simulink model "Ejercicio8"  (R2020a)
settings: Solver=ode15s  StartTime=0.0  StopTime=15  MaxStep=0.012  RelTol=1e-3
values from neighbouring files (symbols this model uses):
  c = 2000    [Ejercicio7_parametros.m]    (also in Ejercicio8_parametros.m)
  k1 = 22000    [Ejercicio8_parametros.m]
  k2 = 10000    [Ejercicio8_parametros.m]
  m1 = 250    [Ejercicio8_parametros.m]
  m2 = 25    [Ejercicio8_parametros.m]
libraries: fl_lib x10, nesl_utility x6, SignalEditorBlockLib x1, sdl_lib x1
settings Model: Creator=juan  LastModifiedBy=juan

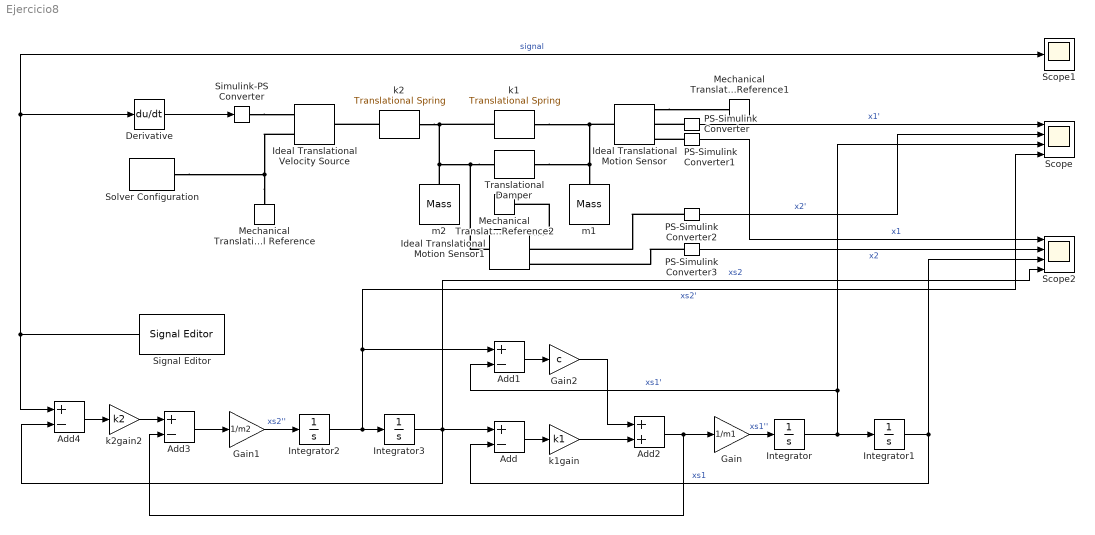
== system Ejercicio8 ==
  Add{,1,3..4} (4 alike) : Sum  Inputs=+-
  Add2 : Sum
  Derivative : Derivative
  Gain : Gain  Gain=1/m1
  Gain1 : Gain  Gain=1/m2
  Gain2 : Gain  Gain=c
  Ideal Translational Motion Sensor : fl_lib/Mechanical/Mechanical Sensors/Ideal Translational Motion Sensor  offset=0 m
  Ideal Translational Motion Sensor1 : fl_lib/Mechanical/Mechanical Sensors/Ideal Translational Motion Sensor  offset=0 m
  Ideal Translational Velocity Source : fl_lib/Mechanical/Mechanical Sources/Ideal Translational Velocity Source
  Integrator{,1..3} (4 alike) : Integrator
  Mechanical Translational Reference : fl_lib/Mechanical/Translational Elements/Mechanical Translational Reference
  Mechanical Translational Reference1 : fl_lib/Mechanical/Translational Elements/Mechanical Translational Reference
  Mechanical Translational Reference2 : fl_lib/Mechanical/Translational Elements/Mechanical Translational Reference
  PS-Simulink Converter{,1..3} (4 alike) : nesl_utility/PS-Simulink Converter  PhysicalDomain=network_engine_domain  SubClassName=ps_output  LeftPortType=input  RightPortType=output  PseudoPeriodic=off  Frequencies=[]  Unit=inherit  AffineConversion=off
  Scope : Scope  NumInputPorts=4
  Scope1 : Scope
  Scope2 : Scope  NumInputPorts=4
  Signal Editor : SignalEditorBlockLib/Signal Editor  FileName=Ejercicio7_terreno.mat  ActiveScenario=Scenario  ActiveSignal=Signal 1  IsBus=off  OutputBusObjectStr=Bus: BusObject  SampleTime=0  ZeroCross=off  OutputAfterFinalValue=Setting to zero  Unit=inherit  PreserveSignalName=on
  Simulink-PS Converter : nesl_utility/Simulink-PS Converter  PhysicalDomain=network_engine_domain  SubClassName=ps_input  LeftPortType=input  RightPortType=output  PseudoPeriodic=off  Frequencies=[]  NoiseDistribution=none  NoiseParameters=[]  Unit=1  AffineConversion=off  FilteringAndDerivatives=provide  SimscapeFilterOrder=1  InputFilterTimeConstant=0.001  UdotUserProvided=0
  Solver Configuration : nesl_utility/Solver Configuration  PhysicalDomain=network_engine_domain  SubClassName=solver  LeftPortType=input  RightPortType=generic  Tones=[]  Harmonics=[]  SimulateNoise=off  Profile=off  UseLocalSampling=off  EnableSwitchedLinearOptims=on  FrequencyDomain=off  UseCCode=off  RelTol=0.001  AbsTol=1e-06  MinStep=1e-09  ToWorkspace=off  RevertToSquareIcSolve=off  NumHomotopyIterations=100  PhasorMode=off  PhasorModeNumHarmonics=1  DoDC=off  ResidualTolerance=1e-09  UseLocalSolver=off  LocalSolverChoice=NE_BACKWARD_EULER_ADVANCER  LocalSolverSampleTime=0.001  DoFixedCost=off  MaxNonlinIter=3  MaxModeIter=2  LinearAlgebra=auto  EquationFormulation=NE_TIME_EF  DelaysMemoryBudget=1024  AutomaticFiltering=on  FilteringTimeConstant=0.001  PartitionStorageMethod=AS_NEEDED  PartitionMemoryBudget=1024  PartitionMethod=ROBUST
  Translational Damper : sdl_lib/Couplings & Drives/Springs & Dampers/Translational Damper  D=c N/(m/s)  enable_faults=0  b_fault=1e6 N/(m/s)  temporal_fault=0  fault_time=5 s  shock_fault=0  acceleration_limit=100 m/s^2  shock_limit=1  report_fault=1
      settings: SourceProductBaseCode=LD
  k1 : fl_lib/Mechanical/Translational Elements/Translational Spring  spr_rate=k1 N/m  v_specify=off  v_priority=None  v=0 m/s  v_nominal_specify=off  v_nominal_unit=m/s  v_nominal_value=1  f_specify=off  f_priority=None  f=0 N  f_nominal_specify=off  f_nominal_unit=N  f_nominal_value=1  x_specify=off  x_priority=High  x=0 m  x_nominal_specify=off  x_nominal_unit=m  x_nominal_value=1
  k1gain : Gain  Gain=k1
  k2 : fl_lib/Mechanical/Translational Elements/Translational Spring  spr_rate=k2 N/m  v_specify=off  v_priority=None  v=0 m/s  v_nominal_specify=off  v_nominal_unit=m/s  v_nominal_value=1  f_specify=off  f_priority=None  f=0 N  f_nominal_specify=off  f_nominal_unit=N  f_nominal_value=1  x_specify=off  x_priority=High  x=0 m  x_nominal_specify=off  x_nominal_unit=m  x_nominal_value=1
  k2gain2 : Gain  Gain=k2
  m1 : fl_lib/Mechanical/Translational Elements/Mass  mass=m1 kg  v_specify=off  v_priority=High  v=0 m/s  v_nominal_specify=off  v_nominal_unit=m/s  v_nominal_value=1  f_specify=off  f_priority=None  f=0 N  f_nominal_specify=off  f_nominal_unit=N  f_nominal_value=1
  m2 : fl_lib/Mechanical/Translational Elements/Mass  mass=m2 kg  v_specify=off  v_priority=High  v=0 m/s  v_nominal_specify=off  v_nominal_unit=m/s  v_nominal_value=1  f_specify=off  f_priority=None  f=0 N  f_nominal_specify=off  f_nominal_unit=N  f_nominal_value=1
  wires:
  PS-Simulink Converter/1 -> Scope/1  "x1'"
  PS-Simulink Converter2/1 -> Scope/2  "x2'"
  Add2/1 -> Gain/1, Add3/2
  PS-Simulink Converter3/1 -> Scope2/2  "x2"
  Integrator/1 -> Scope/3, Add1/2, Integrator1/1  "xs1'"
  Gain/1 -> Integrator/1  "xs1''"
  Gain2/1 -> Add2/1
  Add1/1 -> Gain2/1
  Add/1 -> k1gain/1
  k1gain/1 -> Add2/2
  Signal Editor/1 -> Add4/1, Scope1/1, Derivative/1  "signal"
  PS-Simulink Converter1/1 -> Scope2/1  "x1"
  Integrator1/1 -> Scope2/3, Add/2  "xs1"
  Gain1/1 -> Integrator2/1  "xs2''"
  Integrator2/1 -> Scope/4, Add1/1, Integrator3/1  "xs2'"
  Integrator3/1 -> Scope2/4, Add4/2, Add/1  "xs2"
  Add4/1 -> k2gain2/1
  Derivative/1 -> Simulink-PS Converter/1
  k2gain2/1 -> Add3/1
  Add3/1 -> Gain1/1
  connections:
  Translational Damper/LConn1 -- Ideal Translational Motion Sensor1/LConn1 -- k1/LConn1 -- k2/RConn1 -- m2/LConn1
  Mechanical Translational Reference/LConn1 -- Ideal Translational Velocity Source/RConn2 -- Solver Configuration/RConn1
  Translational Damper/RConn1 -- k1/RConn1 -- Ideal Translational Motion Sensor/LConn1 -- m1/LConn1
  PS-Simulink Converter3/LConn1 -- Ideal Translational Motion Sensor1/RConn3
  Simulink-PS Converter/RConn1 -- Ideal Translational Velocity Source/RConn1
  Ideal Translational Motion Sensor/RConn1 -- Mechanical Translational Reference1/LConn1
  PS-Simulink Converter2/LConn1 -- Ideal Translational Motion Sensor1/RConn2
  PS-Simulink Converter1/LConn1 -- Ideal Translational Motion Sensor/RConn3
  Ideal Translational Motion Sensor1/RConn1 -- Mechanical Translational Reference2/LConn1
  PS-Simulink Converter/LConn1 -- Ideal Translational Motion Sensor/RConn2
  k2/LConn1 -- Ideal Translational Velocity Source/LConn1
